simulink model "FOSTWIN"  (R2022a)
settings: Solver=FixedStepAuto  StartTime=0.0  StopTime=30  FixedStep=Ts  RelTol=1e-3
values from neighbouring files (symbols this model uses):
  D = (1+2*k*h/(sinh(2*k*h)))*tanh(k*h)    [SIDWaveGenerator.m]
  initTime = 2    [initModels_GUI.m]
  Kt = 0.943    [initModels_GUI.m]
  lpFreqCurrent = 50    [initModels_GUI.m]
  lpFreqVelocity = 50    [initModels_GUI.m]
  maxCurrent = 15    [initModels_GUI.m]
  maxFaultCount = 3    [initModels_GUI.m]
  param1 = 5    [initModels_GUI.m]    (also in starttarget.m = param1New)
  param2 = 5    [initModels_GUI.m]    (also in starttarget.m = param2New)
  param3 = 10    [initModels_GUI.m]    (also in starttarget.m = param3New)
  param4 = 10    [initModels_GUI.m]    (also in starttarget.m = param4New)
  safeDamping = 2.5    [initModels_GUI.m]
  safeTime = 20    [initModels_GUI.m]
  stableTime = 3    [initModels_GUI.m]
  Ts = 1/1000    (= 0.001)    [FOSTWINctrlPost.m]    (also in initModels_GUI.m)
  waveH = 1    [SIDWaveGenerator.m]    (also in initModels_GUI.m = 0.136; starttarget.m = waveHNew)
undefined symbols (not defined in the file or in its folder): control_id_twin4, ctrl2TwinStruct, ctrlParam1, ctrlParam2, ctrlParam3, ctrlParam4, ctrlParamStruct, curAft, curBow, dataID_twin6, param5, paramStruct, pcktID, posFlapAft, posFlapBow, SimStateMsg, state, twin2CtrlStruct
libraries: simulink x48, slrealtimeutilitieslib x24, slrealtimeethercatlib x6, slrealtimeloglib x4, dspstat3 x3, slrealtimeiplib x3, slrealtimetgmanagement x1
(part 2 of 2)

== system FOSTWIN/ouput/Remote/Send UDP Data/BuildDataPckts/BuildSignal14 ==
  SignalNo : Inport
  SignalData : Inport  Port=2
  "Byte Packing " : slrealtimeutilitieslib/Byte Packing  MaskPackedDataType=uint8  MaskUnpackedDataTypes={'uint8','uint8','single'}  MaskAlignment=1
  Data Type Conversion : DataTypeConversion  OutDataTypeStr=uint8  SaturateOnIntegerOverflow=off  RndMeth=Floor
  Enumerated Constant : simulink/Sources/Enumerated Constant  OutDataTypeStr=Enum: pcktID  Value=pcktID.data  SampleTime=inf
  SignalBytes : Outport
  wires:
  Data Type Conversion/1 -> "Byte Packing "/1
  Enumerated Constant/1 -> Data Type Conversion/1
  "Byte Packing "/1 -> SignalBytes/1
  SignalData/1 -> "Byte Packing "/3
  SignalNo/1 -> "Byte Packing "/2

== system FOSTWIN/ouput/Remote/Send UDP Data/BuildDataPckts/BuildSignal15 ==
  SignalNo : Inport
  SignalData : Inport  Port=2
  "Byte Packing " : slrealtimeutilitieslib/Byte Packing  MaskPackedDataType=uint8  MaskUnpackedDataTypes={'uint8','uint8','single'}  MaskAlignment=1
  Data Type Conversion : DataTypeConversion  OutDataTypeStr=uint8  SaturateOnIntegerOverflow=off  RndMeth=Floor
  Enumerated Constant : simulink/Sources/Enumerated Constant  OutDataTypeStr=Enum: pcktID  Value=pcktID.data  SampleTime=inf
  SignalBytes : Outport
  wires:
  SignalNo/1 -> "Byte Packing "/2
  SignalData/1 -> "Byte Packing "/3
  "Byte Packing "/1 -> SignalBytes/1
  Enumerated Constant/1 -> Data Type Conversion/1
  Data Type Conversion/1 -> "Byte Packing "/1

== system FOSTWIN/ouput/Remote/Send UDP Data/BuildDataPckts/BuildSignal16 ==
  SignalNo : Inport
  SignalData : Inport  Port=2
  "Byte Packing " : slrealtimeutilitieslib/Byte Packing  MaskPackedDataType=uint8  MaskUnpackedDataTypes={'uint8','uint8','single'}  MaskAlignment=1
  Data Type Conversion : DataTypeConversion  OutDataTypeStr=uint8  SaturateOnIntegerOverflow=off  RndMeth=Floor
  Enumerated Constant : simulink/Sources/Enumerated Constant  OutDataTypeStr=Enum: pcktID  Value=pcktID.data  SampleTime=inf
  SignalBytes : Outport
  wires:
  Data Type Conversion/1 -> "Byte Packing "/1
  Enumerated Constant/1 -> Data Type Conversion/1
  "Byte Packing "/1 -> SignalBytes/1
  SignalData/1 -> "Byte Packing "/3
  SignalNo/1 -> "Byte Packing "/2

== system FOSTWIN/ouput/Remote/Send UDP Data/BuildDataPckts/BuildSignal17 ==
  SignalNo : Inport
  SignalData : Inport  Port=2
  "Byte Packing " : slrealtimeutilitieslib/Byte Packing  MaskPackedDataType=uint8  MaskUnpackedDataTypes={'uint8','uint8','single'}  MaskAlignment=1
  Data Type Conversion : DataTypeConversion  OutDataTypeStr=uint8  SaturateOnIntegerOverflow=off  RndMeth=Floor
  Enumerated Constant : simulink/Sources/Enumerated Constant  OutDataTypeStr=Enum: pcktID  Value=pcktID.data  SampleTime=inf
  SignalBytes : Outport
  wires:
  Data Type Conversion/1 -> "Byte Packing "/1
  Enumerated Constant/1 -> Data Type Conversion/1
  "Byte Packing "/1 -> SignalBytes/1
  SignalData/1 -> "Byte Packing "/3
  SignalNo/1 -> "Byte Packing "/2

== system FOSTWIN/ouput/Remote/Send UDP Data/BuildDataPckts/BuildSignal18 ==
  SignalNo : Inport
  SignalData : Inport  Port=2
  "Byte Packing " : slrealtimeutilitieslib/Byte Packing  MaskPackedDataType=uint8  MaskUnpackedDataTypes={'uint8','uint8','single'}  MaskAlignment=1
  Data Type Conversion : DataTypeConversion  OutDataTypeStr=uint8  SaturateOnIntegerOverflow=off  RndMeth=Floor
  Enumerated Constant : simulink/Sources/Enumerated Constant  OutDataTypeStr=Enum: pcktID  Value=pcktID.data  SampleTime=inf
  SignalBytes : Outport
  wires:
  SignalNo/1 -> "Byte Packing "/2
  SignalData/1 -> "Byte Packing "/3
  "Byte Packing "/1 -> SignalBytes/1
  Enumerated Constant/1 -> Data Type Conversion/1
  Data Type Conversion/1 -> "Byte Packing "/1

== system FOSTWIN/ouput/Remote/Send UDP Data/BuildDataPckts/BuildSignal2 ==
  SignalNo : Inport
  SignalData : Inport  Port=2
  "Byte Packing " : slrealtimeutilitieslib/Byte Packing  MaskPackedDataType=uint8  MaskUnpackedDataTypes={'uint8','uint8','single'}  MaskAlignment=1
  Data Type Conversion : DataTypeConversion  OutDataTypeStr=uint8  SaturateOnIntegerOverflow=off  RndMeth=Floor
  Enumerated Constant : simulink/Sources/Enumerated Constant  OutDataTypeStr=Enum: pcktID  Value=pcktID.data  SampleTime=inf
  SignalBytes : Outport
  wires:
  SignalNo/1 -> "Byte Packing "/2
  SignalData/1 -> "Byte Packing "/3
  "Byte Packing "/1 -> SignalBytes/1
  Enumerated Constant/1 -> Data Type Conversion/1
  Data Type Conversion/1 -> "Byte Packing "/1

== system FOSTWIN/ouput/Remote/Send UDP Data/BuildDataPckts/BuildSignal3 ==
  SignalNo : Inport
  SignalData : Inport  Port=2
  "Byte Packing " : slrealtimeutilitieslib/Byte Packing  MaskPackedDataType=uint8  MaskUnpackedDataTypes={'uint8','uint8','single'}  MaskAlignment=1
  Data Type Conversion : DataTypeConversion  OutDataTypeStr=uint8  SaturateOnIntegerOverflow=off  RndMeth=Floor
  Enumerated Constant : simulink/Sources/Enumerated Constant  OutDataTypeStr=Enum: pcktID  Value=pcktID.data  SampleTime=inf
  SignalBytes : Outport
  wires:
  Data Type Conversion/1 -> "Byte Packing "/1
  Enumerated Constant/1 -> Data Type Conversion/1
  "Byte Packing "/1 -> SignalBytes/1
  SignalData/1 -> "Byte Packing "/3
  SignalNo/1 -> "Byte Packing "/2

== system FOSTWIN/ouput/Remote/Send UDP Data/BuildDataPckts/BuildSignal4 ==
  SignalNo : Inport
  SignalData : Inport  Port=2
  "Byte Packing " : slrealtimeutilitieslib/Byte Packing  MaskPackedDataType=uint8  MaskUnpackedDataTypes={'uint8','uint8','single'}  MaskAlignment=1
  Data Type Conversion : DataTypeConversion  OutDataTypeStr=uint8  SaturateOnIntegerOverflow=off  RndMeth=Floor
  Enumerated Constant : simulink/Sources/Enumerated Constant  OutDataTypeStr=Enum: pcktID  Value=pcktID.data  SampleTime=inf
  SignalBytes : Outport
  wires:
  SignalNo/1 -> "Byte Packing "/2
  SignalData/1 -> "Byte Packing "/3
  "Byte Packing "/1 -> SignalBytes/1
  Enumerated Constant/1 -> Data Type Conversion/1
  Data Type Conversion/1 -> "Byte Packing "/1

== system FOSTWIN/ouput/Remote/Send UDP Data/BuildDataPckts/BuildSignal5 ==
  SignalNo : Inport
  SignalData : Inport  Port=2
  "Byte Packing " : slrealtimeutilitieslib/Byte Packing  MaskPackedDataType=uint8  MaskUnpackedDataTypes={'uint8','uint8','single'}  MaskAlignment=1
  Data Type Conversion : DataTypeConversion  OutDataTypeStr=uint8  SaturateOnIntegerOverflow=off  RndMeth=Floor
  Enumerated Constant : simulink/Sources/Enumerated Constant  OutDataTypeStr=Enum: pcktID  Value=pcktID.data  SampleTime=inf
  SignalBytes : Outport
  wires:
  SignalNo/1 -> "Byte Packing "/2
  SignalData/1 -> "Byte Packing "/3
  "Byte Packing "/1 -> SignalBytes/1
  Enumerated Constant/1 -> Data Type Conversion/1
  Data Type Conversion/1 -> "Byte Packing "/1

== system FOSTWIN/ouput/Remote/Send UDP Data/BuildDataPckts/BuildSignal6 ==
  SignalNo : Inport
  SignalData : Inport  Port=2
  "Byte Packing " : slrealtimeutilitieslib/Byte Packing  MaskPackedDataType=uint8  MaskUnpackedDataTypes={'uint8','uint8','single'}  MaskAlignment=1
  Data Type Conversion : DataTypeConversion  OutDataTypeStr=uint8  SaturateOnIntegerOverflow=off  RndMeth=Floor
  Enumerated Constant : simulink/Sources/Enumerated Constant  OutDataTypeStr=Enum: pcktID  Value=pcktID.data  SampleTime=inf
  SignalBytes : Outport
  wires:
  Data Type Conversion/1 -> "Byte Packing "/1
  Enumerated Constant/1 -> Data Type Conversion/1
  "Byte Packing "/1 -> SignalBytes/1
  SignalData/1 -> "Byte Packing "/3
  SignalNo/1 -> "Byte Packing "/2

== system FOSTWIN/ouput/Remote/Send UDP Data/BuildDataPckts/BuildSignal7 ==
  SignalNo : Inport
  SignalData : Inport  Port=2
  "Byte Packing " : slrealtimeutilitieslib/Byte Packing  MaskPackedDataType=uint8  MaskUnpackedDataTypes={'uint8','uint8','single'}  MaskAlignment=1
  Data Type Conversion : DataTypeConversion  OutDataTypeStr=uint8  SaturateOnIntegerOverflow=off  RndMeth=Floor
  Enumerated Constant : simulink/Sources/Enumerated Constant  OutDataTypeStr=Enum: pcktID  Value=pcktID.data  SampleTime=inf
  SignalBytes : Outport
  wires:
  SignalNo/1 -> "Byte Packing "/2
  SignalData/1 -> "Byte Packing "/3
  "Byte Packing "/1 -> SignalBytes/1
  Enumerated Constant/1 -> Data Type Conversion/1
  Data Type Conversion/1 -> "Byte Packing "/1

== system FOSTWIN/ouput/Remote/Send UDP Data/BuildDataPckts/BuildSignal8 ==
  SignalNo : Inport
  SignalData : Inport  Port=2
  "Byte Packing " : slrealtimeutilitieslib/Byte Packing  MaskPackedDataType=uint8  MaskUnpackedDataTypes={'uint8','uint8','single'}  MaskAlignment=1
  Data Type Conversion : DataTypeConversion  OutDataTypeStr=uint8  SaturateOnIntegerOverflow=off  RndMeth=Floor
  Enumerated Constant : simulink/Sources/Enumerated Constant  OutDataTypeStr=Enum: pcktID  Value=pcktID.data  SampleTime=inf
  SignalBytes : Outport
  wires:
  Data Type Conversion/1 -> "Byte Packing "/1
  Enumerated Constant/1 -> Data Type Conversion/1
  "Byte Packing "/1 -> SignalBytes/1
  SignalData/1 -> "Byte Packing "/3
  SignalNo/1 -> "Byte Packing "/2

== system FOSTWIN/ouput/Remote/Send UDP Data/BuildDataPckts/BuildSignal9 ==
  SignalNo : Inport
  SignalData : Inport  Port=2
  "Byte Packing " : slrealtimeutilitieslib/Byte Packing  MaskPackedDataType=uint8  MaskUnpackedDataTypes={'uint8','uint8','single'}  MaskAlignment=1
  Data Type Conversion : DataTypeConversion  OutDataTypeStr=uint8  SaturateOnIntegerOverflow=off  RndMeth=Floor
  Enumerated Constant : simulink/Sources/Enumerated Constant  OutDataTypeStr=Enum: pcktID  Value=pcktID.data  SampleTime=inf
  SignalBytes : Outport
  wires:
  SignalNo/1 -> "Byte Packing "/2
  SignalData/1 -> "Byte Packing "/3
  "Byte Packing "/1 -> SignalBytes/1
  Enumerated Constant/1 -> Data Type Conversion/1
  Data Type Conversion/1 -> "Byte Packing "/1

== matlab function FOSTWIN/params/Remote/MATLAB Function ==
  data: error output; busOut output Bus: slBus1; udpData input; busIn input
function [error, busOut] = fcn(udpData, busIn)

numPcktBytes = 6;

busOut = busIn;
error = 0;
%if we haven't gotten a new command in 
if size(udpData) == 0
    return
end


if mod(size(udpData),numPcktBytes) ~= 0
    error = 1;
    return
end

if size(udpData) < numPcktBytes
    error = 2;
    return
end

headerID = udpData(1);
if headerID ~= 1
    error = 3;
    return
end

payloadSize = udpData(2);
if size(udpData) ~= numPcktBytes + payloadSize * numPcktBytes
    error = 4;
    return
end

for n=1:payloadSize
   
    baseIndex = numPcktBytes + (n-1)*numPcktBytes;
    
    dataID = udpData(baseIndex + 1);
    
    if dataID ~= 4 % dataId of 4 means param packet (7th index of byte array sent in) 
        error = 5;
        return
    end
    
    dataType = paramTypeEnum_Twin_v4(udpData(baseIndex + 2));
    
    dataData = typecast(udpData(baseIndex + 3: baseIndex+6)  , 'single');
    
    switch dataType
        case paramTypeEnum_Twin_v4.setParam1
            busOut.param1 = double(dataData);
        case paramTypeEnum_Twin_v4.setParam2
            busOut.param2 = double(dataData);
        case paramTypeEnum_Twin_v4.setParam3
            busOut.param3 = double(dataData); % developer will need to convert double 0/1 to logical in their model
        case paramTypeEnum_Twin_v4.setParam4
            busOut.param4 = double(dataData);
        case paramTypeEnum_Twin_v4.setParam5
            busOut.param5 = double(dataData); % waveHeight
        otherwise
            % nothing here
    end
end

== stateflow chart FOSTWIN/stateCtrl/Chart ==
  state init
    entry:
    state = fostwinStateEnum.init;
    faultCount = 0;
    during:
    bowCurrentOut = 0;
    aftCurrentOut = 0;
  note: This wait time is representative for a controller booting up for a real machine.
  state normal
    entry:
    state = fostwinStateEnum.ctrlNormal;
    during:
    bowCurrentOut = bowCurrentRawIn;
    aftCurrentOut = aftCurrentRawIn;
  state stabilize
    entry:
    state = fostwinStateEnum.ctrlStabilize;
    faultCount = faultCount + 1;
    during:
    bowCurrentOut = 0;
    aftCurrentOut = 0;
  state ctrlSafe
    entry:
    state = fostwinStateEnum.ctrlSafe;
    during:
    bowCurrentOut = - safeDamping * bowVelocity / Kt;
    aftCurrentOut = - safeDamping * aftVelocity / Kt;
  state ctrtFault
    entry:
    state = fostwinStateEnum.ctrlFault;
    during:
    bowCurrentOut = 0;
    aftCurrentOut = 0;
  (default) -> init
  init -> normal : [after(initTime,'sec')]
  ctrlSafe -> normal [order 2] : [after(safeTime, 'sec')]
  normal -> stabilize : [abs(bowCurrentFilteredIn) >= maxCurrent || ...
      | abs(aftCurrentFilteredIn) >= maxCurrent]
  stabilize -> ctrtFault [order 1] : [faultCount >= maxFaultCount]
  stabilize -> ctrlSafe [order 2] : [after(stableTime,'sec')]
  ctrlSafe -> stabilize [order 1] : [abs(bowCurrentFilteredIn) >= maxCurrent || ...
      | abs(aftCurrentFilteredIn) >= maxCurrent]
  data: aftCurrentRawIn input; bowCurrentRawIn input; aftCurrentFilteredIn input; bowCurrentFilteredIn input; state output Enum: fostwinStateEnum size=1; aftCurrentOut output; bowCurrentOut output; Kt parameter; safeDamping parameter; safeTime parameter; maxCurrent parameter; aftVelocity input; bowVelocity input; maxFaultCount parameter; faultCount local; stableTime parameter; initTime parameter
